simulink model "final_project_model"  (R2015b)
settings: Solver=VariableStepAuto  StartTime=0.0  StopTime=12  RelTol=1e-3
values from neighbouring files (symbols this model uses):
  A = .00004264    (= 4.264e-05)    [final_project.m]
  ain = 70    [final_project.m]
  aout = 90    [final_project.m]
  B = .0002100    (= 0.00021)    [final_project.m]
  C = .0002357    (= 0.0002357)    [final_project.m]
  cap = 19.6347222    [final_project.m]
  Kd = 24    [final_project.m]
  Ki = 4    [final_project.m]
  kout = 0.4824    [final_project.m]
  Kp = 8000    [final_project.m]
  qin = 6.6840278    [final_project.m]
settings Model: Creator=Class2019  LastModifiedBy=Class2019

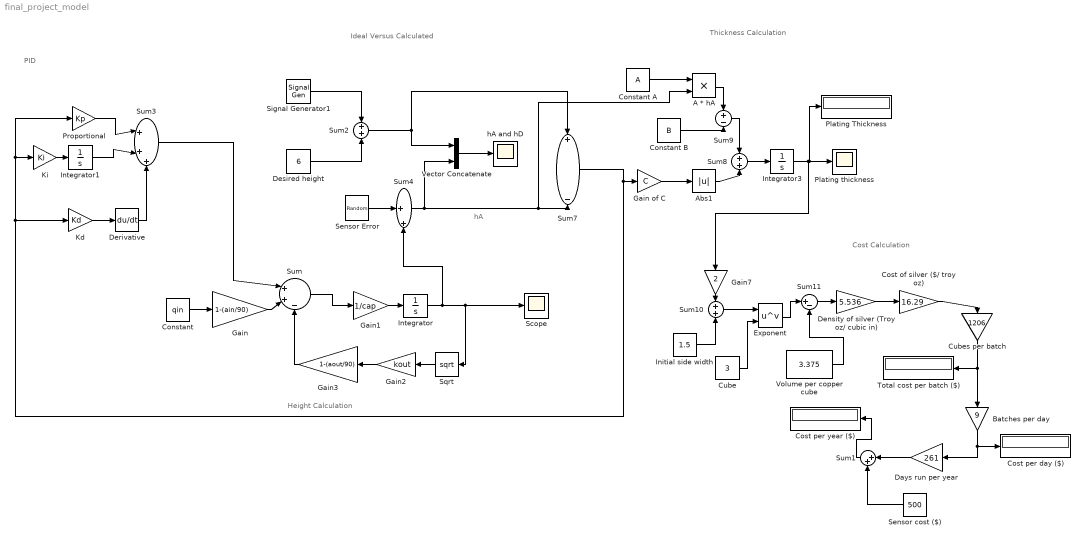
== system final_project_model ==
  note: Ideal Versus Calculated
  note: Height Calculation
  note: Thickness Calculation
  note: Cost Calculation
  note: PID
  note: hA
  A * hA : Product
  Abs1 : Abs
  Batches per day : Gain  Gain=9
  Constant : Constant  Value=qin
  Constant A : Constant  Value=A
  Constant B : Constant  Value=B
  Cost of silver ($/ troy oz) : Gain  Gain=16.29
  Cost per day ($) : Display
  Cost per year ($) : Display
  "Cube " : Constant  Value=3
  Cubes per batch : Gain  Gain=1206
  Days run per year : Gain  Gain=261
  Density of silver (Troy oz/ cubic in) : Gain  Gain=5.536
  Derivative : Derivative
  Desired height : Constant  Value=6
  "Exponent " : Math  Operator=pow  SaturateOnIntegerOverflow=on
  Gain : Gain  Gain=1-(ain/90)
  Gain of C : Gain  Gain=C
  Gain1 : Gain  Gain=1/cap
  Gain2 : Gain  Gain=kout
  Gain3 : Gain  Gain=1-(aout/90)
  Gain7 : Gain  Gain=2
  "Initial side width " : Constant  Value=1.5
  Integrator : Integrator  InitialCondition=6
  Integrator1 : Integrator
  Integrator3 : Integrator
  Kd : Gain  Gain=Kd
  Ki : Gain  Gain=Ki
  "Plating Thickness " : Display
  "Plating thickness " : Scope
  Proportional : Gain  Gain=Kp
  Scope : Scope
  Sensor Error : UniformRandomNumber  Minimum=-.1969/12  Maximum=.1969/12  Seed=8  SampleTime=0.1
  Sensor cost ($) : Constant  Value=500
  Signal Generator1 : SignalGenerator  Amplitude=(.25*2)/12  Frequency=1/2
  Sqrt : Sqrt  SaturateOnIntegerOverflow=on
  Sum : Sum  Inputs=|++-
  Sum1 : Sum  Inputs=|++
  Sum10 : Sum
  Sum11 : Sum  Inputs=|+-
  Sum2 : Sum
  Sum3 : Sum  Inputs=|+++
  Sum4 : Sum  Inputs=|++
  Sum7 : Sum  Inputs=+-
  Sum8 : Sum
  Sum9 : Sum  Inputs=+-
  Total cost per batch ($) : Display
  Vector Concatenate : Concatenate
  "Volume per copper cube " : Constant  Value=3.375
  hA and hD : Scope
  wires:
  Constant/1 -> Gain/1
  Gain1/1 -> Integrator/1
  Integrator/1 -> Scope/1, Sqrt/1, Sum4/2
  Sqrt/1 -> Gain2/1
  Gain2/1 -> Gain3/1
  Sum/1 -> Gain1/1
  Gain3/1 -> Sum/3
  Proportional/1 -> Sum3/1
  Integrator1/1 -> Sum3/2
  Ki/1 -> Integrator1/1
  Derivative/1 -> Sum3/3
  Kd/1 -> Derivative/1
  Signal Generator1/1 -> Sum2/1
  Desired height/1 -> Sum2/2
  Vector Concatenate/1 -> hA and hD/1
  Sum2/1 -> Sum7/1, Vector Concatenate/1
  Gain/1 -> Sum/2
  Sensor Error/1 -> Sum4/1
  Sum4/1 -> A * hA/2, Sum7/2, Vector Concatenate/2
  Sum3/1 -> Sum/1
  Sum7/1 -> Proportional/1, Ki/1, Kd/1, Gain of C/1
  Gain of C/1 -> Abs1/1
  Abs1/1 -> Sum8/2
  Sum9/1 -> Sum8/1
  Constant B/1 -> Sum9/2
  A * hA/1 -> Sum9/1
  Constant A/1 -> A * hA/1
  Sum8/1 -> Integrator3/1
  Integrator3/1 -> "Plating Thickness "/1, "Plating thickness "/1, Gain7/1
  Gain7/1 -> Sum10/1
  "Initial side width "/1 -> Sum10/2
  Sum10/1 -> "Exponent "/1
  "Cube "/1 -> "Exponent "/2
  "Exponent "/1 -> Sum11/1
  "Volume per copper cube "/1 -> Sum11/2
  Sum11/1 -> Density of silver (Troy oz/ cubic in)/1
  Density of silver (Troy oz/ cubic in)/1 -> Cost of silver ($/ troy oz)/1
  Cost of silver ($/ troy oz)/1 -> Cubes per batch/1
  Cubes per batch/1 -> Batches per day/1, Total cost per batch ($)/1
  Batches per day/1 -> Cost per day ($)/1, Days run per year/1
  Days run per year/1 -> Sum1/1
  Sensor cost ($)/1 -> Sum1/2
  Sum1/1 -> Cost per year ($)/1
